simulink model "PI"  (R2020b)
settings: Solver=VariableStepAuto  StartTime=0.0  StopTime=10.0  RelTol=1e-3
undefined symbols (not defined in the file or in its folder): Kd, Ki, Kp, N
settings Model: DataDictionary=cruise_model_cum_controller_parametrs.sldd  Creator=153  LastModifiedBy=153
settings DataIOCC: SaveOutput=off  SaveTime=off

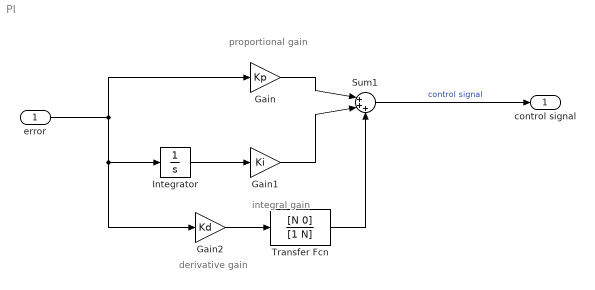
== system PI ==
  note: derivative gain
  note: proportional gain
  note: integral gain
  error : Inport  OutDataTypeStr=double  PortDimensions=1  SampleTime=0
  Gain : Gain  Gain=Kp
  Gain1 : Gain  Gain=Ki
  Gain2 : Gain  Gain=Kd
  Integrator : Integrator
  Sum1 : Sum  Inputs=|+++
  Transfer Fcn : TransferFcn  Numerator=[N 0]  Denominator=[1 N]
  control signal : Outport  OutDataTypeStr=double  PortDimensions=1  SampleTime=0
  wires:
  Integrator/1 -> Gain1/1
  error/1 -> Gain/1, Gain2/1, Integrator/1
  Gain/1 -> Sum1/1
  Gain1/1 -> Sum1/2
  Sum1/1 -> control signal/1  "control signal"
  Gain2/1 -> Transfer Fcn/1
  Transfer Fcn/1 -> Sum1/3
